simulink model "MIMOOFDMfinal2"  (Simulink 7.5)
settings: Solver=ode45  StartTime=0.0  StopTime=5000  RelTol=1e-3
StartFcn:
  | global Pi;
  | global ber;
  | Pi=[0;0;0;0];
  | ber=0;
libraries: dspbuff3 x8, dspxfrm3 x6, dspmtrx3 x1, commrandsrc2 x1
settings Model: Creator=him  LastModifiedBy=him

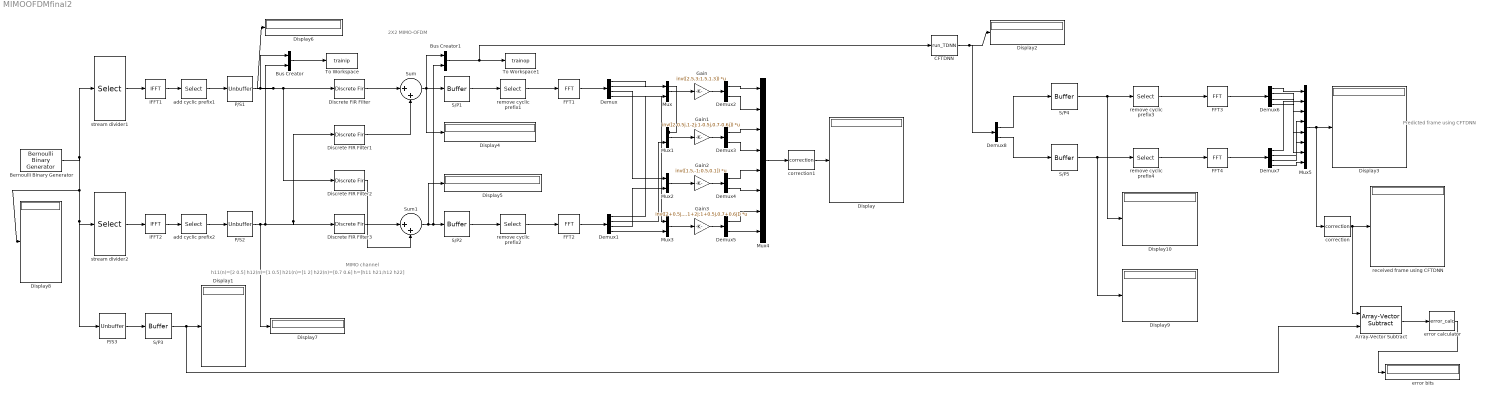
== system MIMOOFDMfinal2 ==
  note: MIMO channel
  note: 2X2 MIMO-OFDM
  note: h11(n)=[2 0.5]
      | h12(n)=[1 0.5]
      | h21(n)=[1 2]
      | h22(n)=[0.7 0.6]
      |
      | h=[h11 h21;h12 h22]
  note: Predicted frame
      | using
      | CFTDNN
  Array-Vector Subtract : dspmtrx3/Array-Vector Subtract  DialogController=dspDDGCreate  DialogControllerArgs=DataTag0  Dimension=1  V_Source=Input port  V_VectFromMask=[0.5 0.25]  firstCoeffDataTypeStr=Inherit: Same word length as input  firstCoeffLastDataTypeStr=Inherit: Same word length as input  firstCoeffMin=[]  firstCoeffMax=[]  outputDataTypeStr=Inherit: Same as accumulator  outputLastDataTypeStr=Inherit: Same as accumulator  outputMin=[]  outputMax=[]  roundingMode=Floor  overflowMode=off
  Bernoulli Binary Generator : commrandsrc2/Bernoulli Binary Generator  DialogController=commDDGCreate  DialogControllerArgs=DataTag1  SystemSampleTime=-1  P=0.5  seed=61  Ts=1  frameBased=on  sampPerFrame=8  orient=off  outDataType=double
  Bus Creator : BusCreator  Inputs=2
  Bus Creator1 : BusCreator  Inputs=2
  CFTDNN : MATLABFcn  MATLABFcn=run_TDNN  Output1D=off
  Demux{,1,6..7} (4 alike) : Demux
  Demux{2..5,8} (5 alike) : Demux  Outputs=2
  Discrete FIR Filter : DiscreteFir  NumCoeffs=[2 0.5]
  Discrete FIR Filter1 : DiscreteFir  NumCoeffs=[1 2]
  Discrete FIR Filter2 : DiscreteFir  NumCoeffs=[1 0.5]
  Discrete FIR Filter3 : DiscreteFir  NumCoeffs=[0.7 0.6]
  Display{,1..10} (11 alike) : Display
  FFT1 : dspxfrm3/FFT  DialogController=dspDDGCreate  DialogControllerArgs=DataTag2  CompMethod=Table lookup  TableOpt=NEW  TableOptActive=Speed  BitRevOrder=off  InheritFFTLength=on  FFTLength=64  SkipNorm=off  firstCoeffDataTypeStr=Inherit: Same word length as input  firstCoeffLastDataTypeStr=Inherit: Same word length as input  outputMin=[]  outputMax=[]  roundingMode=Floor  overflowMode=off
  FFT2 : dspxfrm3/FFT  DialogController=dspDDGCreate  DialogControllerArgs=DataTag3  CompMethod=Table lookup  TableOpt=NEW  TableOptActive=Speed  BitRevOrder=off  InheritFFTLength=on  FFTLength=64  SkipNorm=off  firstCoeffDataTypeStr=Inherit: Same word length as input  firstCoeffLastDataTypeStr=Inherit: Same word length as input  outputMin=[]  outputMax=[]  roundingMode=Floor  overflowMode=off
  FFT3 : dspxfrm3/FFT  DialogController=dspDDGCreate  DialogControllerArgs=DataTag4  CompMethod=Table lookup  TableOpt=NEW  TableOptActive=Speed  BitRevOrder=off  InheritFFTLength=on  FFTLength=64  SkipNorm=off  firstCoeffDataTypeStr=Inherit: Same word length as input  firstCoeffLastDataTypeStr=Inherit: Same word length as input  outputMin=[]  outputMax=[]  roundingMode=Floor  overflowMode=off
  FFT4 : dspxfrm3/FFT  DialogController=dspDDGCreate  DialogControllerArgs=DataTag5  CompMethod=Table lookup  TableOpt=NEW  TableOptActive=Speed  BitRevOrder=off  InheritFFTLength=on  FFTLength=64  SkipNorm=off  firstCoeffDataTypeStr=Inherit: Same word length as input  firstCoeffLastDataTypeStr=Inherit: Same word length as input  outputMin=[]  outputMax=[]  roundingMode=Floor  overflowMode=off
  Gain : Gain  Gain=inv([2.5,3;1.5,1.3])  Multiplication=Matrix(K*u)  ParameterDataType=fixdt(1, 16)  ParameterScaling=2^0  OutDataType=fixdt(1, 16)  OutScaling=2^0
  Gain1 : Gain  Gain=inv([2-0.5j,1-2j;1-0.5j,0.7-0.6j])  Multiplication=Matrix(K*u)  ParameterDataType=fixdt(1, 16)  ParameterScaling=2^0  OutDataType=fixdt(1, 16)  OutScaling=2^0
  Gain2 : Gain  Gain=inv([1.5,-1;0.5,0.1])  Multiplication=Matrix(K*u)  ParameterDataType=fixdt(1, 16)  ParameterScaling=2^0  OutDataType=fixdt(1, 16)  OutScaling=2^0
  Gain3 : Gain  Gain=inv([2+0.5j,1+2j;1+0.5j,0.7+0.6j])  Multiplication=Matrix(K*u)  ParameterDataType=fixdt(1, 16)  ParameterScaling=2^0  OutDataType=fixdt(1, 16)  OutScaling=2^0
  IFFT1 : dspxfrm3/IFFT  DialogController=dspDDGCreate  DialogControllerArgs=DataTag6  CompMethod=Table lookup  TableOpt=NEW  TableOptActive=Speed  BitRevOrder=off  cs_in=off  SkipNorm=on  InheritFFTLength=on  FFTLength=64  mode=Complex  outSamplingMode=Frame based  firstCoeffDataTypeStr=Inherit: Same word length as input  firstCoeffLastDataTypeStr=Inherit: Same word length as input  outputMin=[]  outputMax=[]  roundingMode=Floor  overflowMode=off
  IFFT2 : dspxfrm3/IFFT  DialogController=dspDDGCreate  DialogControllerArgs=DataTag7  CompMethod=Table lookup  TableOpt=NEW  TableOptActive=Speed  BitRevOrder=off  cs_in=off  SkipNorm=on  InheritFFTLength=on  FFTLength=64  mode=Complex  outSamplingMode=Frame based  firstCoeffDataTypeStr=Inherit: Same word length as input  firstCoeffLastDataTypeStr=Inherit: Same word length as input  outputMin=[]  outputMax=[]  roundingMode=Floor  overflowMode=off
  Mux{,1..3} (4 alike) : Mux  Inputs=2
  Mux4 : Mux  Inputs=8
  Mux5 : Mux  Inputs=8
  P/S1 : dspbuff3/Unbuffer  ic=0
  P/S2 : dspbuff3/Unbuffer  ic=0
  P/S3 : dspbuff3/Unbuffer  ic=0
  S/P{1..2,4..5} (4 alike) : dspbuff3/Buffer  N=5  V=0  ic=0
  S/P3 : dspbuff3/Buffer  N=8  V=0  ic=0
  Sum : Sum  Inputs=|++  OutDataType=fixdt(1, 16)  OutScaling=2^0
  Sum1 : Sum  Inputs=|++  OutDataType=fixdt(1, 16)  OutScaling=2^0
  To Workspace : ToWorkspace  VariableName=trainip  SampleTime=-1  SaveFormat=Array
  To Workspace1 : ToWorkspace  VariableName=trainop  SampleTime=-1  SaveFormat=Array
  add cyclic prefix1 : Selector  InputPortWidth=4  IndexOptions=Index vector (dialog)  Indices=[4,1:4]  OutputSizes=1
  add cyclic prefix2 : Selector  InputPortWidth=4  IndexOptions=Index vector (dialog)  Indices=[4,1:4]  OutputSizes=1
  correction : MATLABFcn  MATLABFcn=correction  Output1D=off
  correction1 : MATLABFcn  MATLABFcn=correction  Output1D=off
  error bits : Display
  error calculator : MATLABFcn  MATLABFcn=error_calc  Output1D=off
  received frame using CFTDNN : Display
  remove cyclic prefix{1..4} (4 alike) : Selector  InputPortWidth=5  IndexOptions=Index vector (dialog)  Indices=[2:5]  OutputSizes=1
  stream divider1 : Selector  InputPortWidth=8  IndexOptions=Index vector (dialog)  Indices=[1,3,5,7]  OutputSizes=1
  stream divider2 : Selector  InputPortWidth=8  IndexOptions=Index vector (dialog)  Indices=[2,4,6,8]  OutputSizes=1
  wires:
  IFFT1/1 -> add cyclic prefix1/1
  add cyclic prefix1/1 -> P/S1/1
  S/P1/1 -> remove cyclic prefix1/1
  remove cyclic prefix1/1 -> FFT1/1
  stream divider1/1 -> IFFT1/1
  IFFT2/1 -> add cyclic prefix2/1
  add cyclic prefix2/1 -> P/S2/1
  stream divider2/1 -> IFFT2/1
  Discrete FIR Filter/1 -> Sum/1
  Discrete FIR Filter1/1 -> Sum/2
  P/S1/1 -> Bus Creator/1, Discrete FIR Filter2/1, Discrete FIR Filter/1, Display6/1
  P/S2/1 -> Bus Creator/2, Discrete FIR Filter1/1, Discrete FIR Filter3/1, Display7/1
  Discrete FIR Filter2/1 -> Sum1/2
  Discrete FIR Filter3/1 -> Sum1/1
  S/P2/1 -> remove cyclic prefix2/1
  remove cyclic prefix2/1 -> FFT2/1
  Sum/1 -> S/P1/1, Bus Creator1/1, Display4/1
  Sum1/1 -> S/P2/1, Bus Creator1/2, Display5/1
  FFT1/1 -> Demux/1
  FFT2/1 -> Demux1/1
  Mux/1 -> Gain/1
  Mux1/1 -> Gain1/1
  Mux2/1 -> Gain2/1
  Mux3/1 -> Gain3/1
  Demux/1 -> Mux/1
  Demux1/1 -> Mux/2
  Demux/2 -> Mux1/1
  Demux1/2 -> Mux1/2
  Demux/3 -> Mux2/1
  Demux1/3 -> Mux2/2
  Demux/4 -> Mux3/1
  Demux1/4 -> Mux3/2
  Gain/1 -> Demux2/1
  Gain1/1 -> Demux3/1
  Demux2/1 -> Mux4/1
  Demux2/2 -> Mux4/2
  Demux3/1 -> Mux4/3
  Demux3/2 -> Mux4/4
  Demux4/1 -> Mux4/5
  Demux4/2 -> Mux4/6
  Demux5/1 -> Mux4/7
  Demux5/2 -> Mux4/8
  Gain3/1 -> Demux5/1
  Gain2/1 -> Demux4/1
  Bus Creator/1 -> To Workspace/1
  Bus Creator1/1 -> To Workspace1/1, CFTDNN/1
  CFTDNN/1 -> Display2/1, Demux8/1
  Bernoulli Binary Generator/1 -> stream divider1/1, Display8/1, stream divider2/1, P/S3/1
  P/S3/1 -> S/P3/1
  S/P3/1 -> Display1/1, Array-Vector Subtract/2
  Demux8/2 -> S/P5/1
  Demux8/1 -> S/P4/1
  S/P5/1 -> remove cyclic prefix4/1, Display9/1
  S/P4/1 -> remove cyclic prefix3/1, Display10/1
  remove cyclic prefix3/1 -> FFT3/1
  remove cyclic prefix4/1 -> FFT4/1
  FFT4/1 -> Demux7/1
  FFT3/1 -> Demux6/1
  Demux7/4 -> Mux5/8
  Demux6/4 -> Mux5/7
  Demux7/3 -> Mux5/6
  Demux6/3 -> Mux5/5
  Demux7/2 -> Mux5/4
  Demux6/2 -> Mux5/3
  Demux7/1 -> Mux5/2
  Demux6/1 -> Mux5/1
  Mux5/1 -> Display3/1, correction/1
  correction/1 -> received frame using CFTDNN/1, Array-Vector Subtract/1
  Mux4/1 -> correction1/1
  correction1/1 -> Display/1
  Array-Vector Subtract/1 -> error calculator/1
  error calculator/1 -> error bits/1
